simulink library "signUnitConverters"  (R2015b)
settings: Solver=VariableStepAuto  StartTime=0.0  StopTime=10.0  RelTol=1e-3
undefined symbols (not defined in the file or in its folder): tireRadius
settings Model: Creator=hyong  LastModifiedBy=hyong

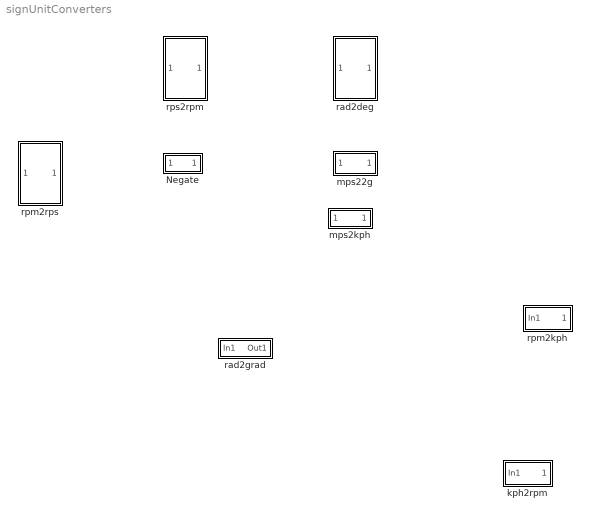
== system signUnitConverters ==
  Negate : Subsystem
  kph2rpm : Subsystem
  mps22g : Subsystem
  mps2kph : Subsystem
  rad2deg : Subsystem
  rad2grad : Subsystem
  rpm2kph : Subsystem
  rpm2rps : Subsystem  AncestorBlock=signUnitConverters/rps2rpm
      settings: OpenFcn=mylib
  rps2rpm : Subsystem
      settings: OpenFcn=mylib

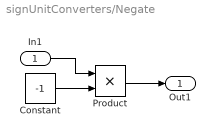
== system signUnitConverters/Negate ==
  In1 : Inport
  Constant : Constant  Value=-1
  Product : Product
  Out1 : Outport
  wires:
  Product/1 -> Out1/1
  In1/1 -> Product/1
  Constant/1 -> Product/2

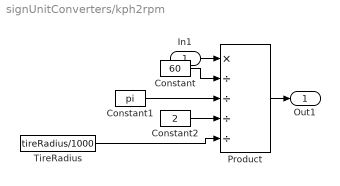
== system signUnitConverters/kph2rpm ==
  In1 : Inport
  Constant : Constant  Value=60
  Constant1 : Constant  Value=pi
  Constant2 : Constant  Value=2
  Product : Product  Inputs=*////
  TireRadius : Constant  Value=tireRadius/1000
  Out1 : Outport
  wires:
  Constant1/1 -> Product/3
  TireRadius/1 -> Product/5
  Constant2/1 -> Product/4
  Constant/1 -> Product/2
  In1/1 -> Product/1
  Product/1 -> Out1/1

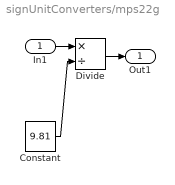
== system signUnitConverters/mps22g ==
  In1 : Inport
  Constant : Constant  Value=9.81
  Divide : Product  Inputs=*/
  Out1 : Outport
  wires:
  Divide/1 -> Out1/1
  In1/1 -> Divide/1
  Constant/1 -> Divide/2

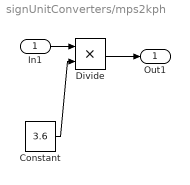
== system signUnitConverters/mps2kph ==
  In1 : Inport
  Constant : Constant  Value=3.6
  Divide : Product  Inputs=**
  Out1 : Outport
  wires:
  In1/1 -> Divide/1
  Constant/1 -> Divide/2
  Divide/1 -> Out1/1

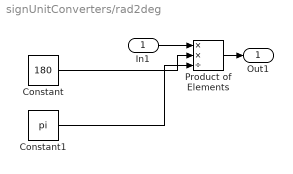
== system signUnitConverters/rad2deg ==
  In1 : Inport
  Constant : Constant  Value=180
  Constant1 : Constant  Value=pi
  Product of Elements : Product  Inputs=**/
  Out1 : Outport
  wires:
  Constant/1 -> Product of Elements/2
  In1/1 -> Product of Elements/1
  Constant1/1 -> Product of Elements/3
  Product of Elements/1 -> Out1/1

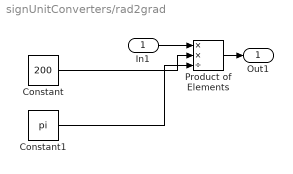
== system signUnitConverters/rad2grad ==
  In1 : Inport
  Constant : Constant  Value=200
  Constant1 : Constant  Value=pi
  Product of Elements : Product  Inputs=**/
  Out1 : Outport
  wires:
  Product of Elements/1 -> Out1/1
  Constant1/1 -> Product of Elements/3
  In1/1 -> Product of Elements/1
  Constant/1 -> Product of Elements/2

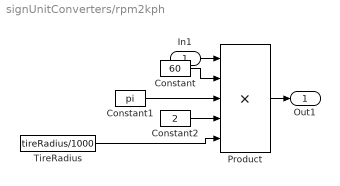
== system signUnitConverters/rpm2kph ==
  In1 : Inport
  Constant : Constant  Value=60
  Constant1 : Constant  Value=pi
  Constant2 : Constant  Value=2
  Product : Product  Inputs=*****
  TireRadius : Constant  Value=tireRadius/1000
  Out1 : Outport
  wires:
  Constant1/1 -> Product/3
  TireRadius/1 -> Product/5
  Constant2/1 -> Product/4
  Constant/1 -> Product/2
  In1/1 -> Product/1
  Product/1 -> Out1/1

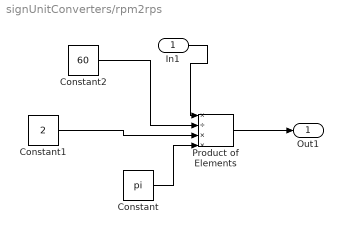
== system signUnitConverters/rpm2rps ==
  In1 : Inport
  Constant : Constant  Value=pi
  Constant1 : Constant  Value=2
  Constant2 : Constant  Value=60
  Product of Elements : Product  Inputs=*/**
  Out1 : Outport
  wires:
  Constant1/1 -> Product of Elements/3
  Product of Elements/1 -> Out1/1
  Constant2/1 -> Product of Elements/2
  In1/1 -> Product of Elements/1
  Constant/1 -> Product of Elements/4

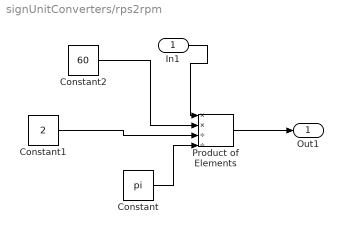
== system signUnitConverters/rps2rpm ==
  In1 : Inport
  Constant : Constant  Value=pi
  Constant1 : Constant  Value=2
  Constant2 : Constant  Value=60
  Product of Elements : Product  Inputs=**//
  Out1 : Outport
  wires:
  Constant1/1 -> Product of Elements/3
  Product of Elements/1 -> Out1/1
  Constant2/1 -> Product of Elements/2
  In1/1 -> Product of Elements/1
  Constant/1 -> Product of Elements/4
